simulink model "generate_joint_position_motion"  (R2021a)
settings: Solver=FixedStepDiscrete  StartTime=0.0  StopTime=inf  FixedStep=0.001  RelTol=1e-3  EnableMultiTasking=on
PreLoadFcn:
  | demos_common_configs();
libraries: franka_simulink_library x5, franka_simulink_library_misc x5
settings Model: SimulationMode=external  ExtModeTrigDuration=10000  Creator=vasi_ko  LastModifiedBy=kvasios
settings SolverCC: AlgebraicLoopSolver=TrustRegion
settings DataIOCC: LimitDataPoints=on  SaveFormat=Array  ReturnWorkspaceOutputs=off
settings OptimizationCC: DefaultParameterBehavior=Inlined  EnhancedBackFolding=on  PassReuseOutputArgsAs=Individual arguments  ZeroExternalMemoryAtStartup=off  ZeroInternalMemoryAtStartup=off  OptimizeBlockOrder=speed  DifferentSizesBufferReuse=on  OptimizationCustomize=off  EfficientTunableParamExpr=on
settings DebuggingCC: SolverPrmCheckMsg=warning  ParameterTunabilityLossMsg=error  SFUnexpectedBacktrackingDiag=warning  SFNoUnconditionalDefaultTransitionDiag=warning  SFExecutionAtInitializationDiag=none  SFMachineParentedDataDiag=warning  ArithmeticOperatorsInVariantConditions=warning
settings HardwareCC: ProdBitPerLong=64  ProdHWDeviceType=Intel->x86-64 (Linux 64)
settings ModelReferenceCC: PropagateSignalLabelsOutOfModel=off
settings SFSimCC: SimUseLocalCustomCode=off  MATLABDynamicMemAlloc=off  CustomCodeUndefinedFunction=UseInterfaceOnly  SimTargetLang=C++
settings RTWCC: SystemTargetFile=franka_emika_panda.tlc  GenCodeOnly=on  TemplateMakefile=ert_default_tmf  RTWVerbose=off  RTWUseLocalCustomCode=off  Toolchain=Franka Simulink | gmake (64-bit linux)  BuildConfiguration=Faster Runs  IncludeHyperlinkInReport=on  TargetLang=C++
settings CodeAppCC: ForceParamTrailComments=on  IgnoreCustomStorageClasses=off  OperatorAnnotations=on  SimulinkDataObjDesc=on  SFDataObjDesc=on  InsertBlockDesc=on
settings STFCustomTargetCC: TargetLangStandard=C99 (ISO)  MultiwordLength=256  GenerateSampleERTMain=on  ModelReferenceCompliant=off  CombineOutputUpdateFcns=on  ERTCustomFileBanners=on  SupportNonInlinedSFcns=off  RemoveResetFunc=on  MATLABClassNameForMDSCustomization=Simulink.SoftwareTarget.ERTCustomization  CPPClassGenCompliant=on  GRTInterface=off  SystemTargetFile=franka_emika_panda.tlc
settings ERTTargetCC: TargetLangStandard=C99 (ISO)  GenerateSampleERTMain=on  ModelReferenceCompliant=off  ParMdlRefBuildCompliant=off  CompOptLevelCompliant=off  ConcurrentExecutionCompliant=off  SupportContinuousTime=on  ModelStepFunctionPrototypeControlCompliant=off  InlinedParameterPlacement=NonHierarchical  ERTCustomFileTemplate=franka_emika_panda_file_process.tlc
settings ConfigComp: CovMetricSettings=dw  CovSaveCumulativeToWorkspaceVar=on  CovSaveSingleToWorkspaceVar=on  CovExternalEMLEnable=off  CovSFcnEnable=off

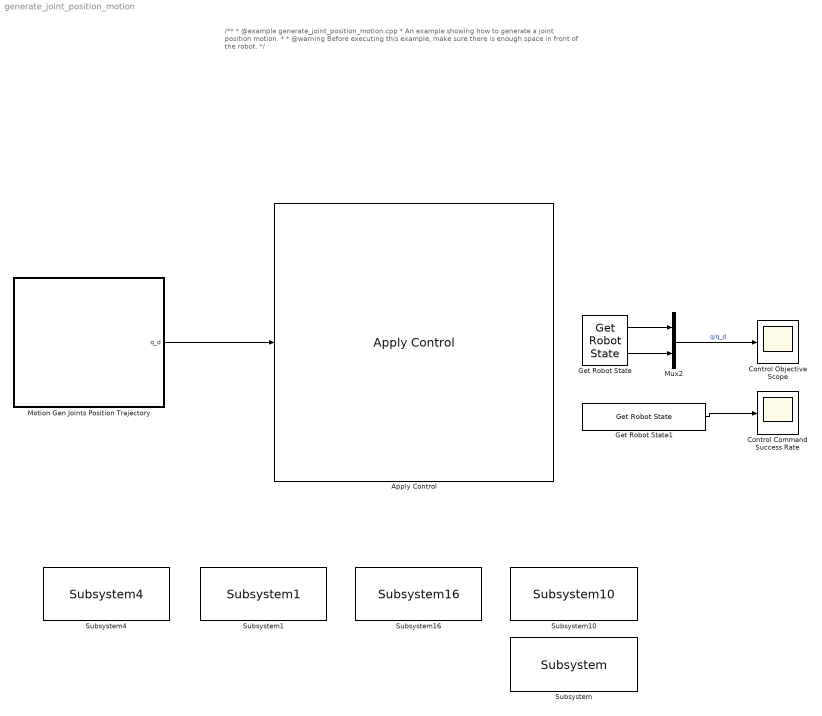
== system generate_joint_position_motion ==
  note: /**
      |  * @example generate_joint_position_motion.cpp
      |  * An example showing how to generate a joint position motion.
      |  *
      |  * @warning Before executing this example, make sure there is enough space in front of the robot.
      |  */
  Apply Control : franka_simulink_library/Apply Control  robot_ip=robot_ip  gripper_attached=off  control_mode=Joint Positions - Internal Controller Mode  controller_choice=Joint Impedance Controller  elbow_control=on  collision_thresholds=collision_behavior  joint_impedance=joint_impedance  cartesian_impedance=cartesian_impedance  load_inertia=load_inertia  EE_T_K=EE_T_K  init_joint_configuration_req=on  init_joint_configuration=q_init
      settings: SourceProductName=Franka Emika
  Control Command Success Rate : Scope
  Control Objective Scope : Scope
  Get Robot State : franka_simulink_library/Get Robot State  robot_ip=robot_ip  signals_requested='q q_d'
      settings: SourceProductName=Franka Emika
  Get Robot State1 : franka_simulink_library/Get Robot State  robot_ip=robot_ip  signals_requested='control_command_success_rate'
      settings: SourceProductName=Franka Emika
  Motion Gen Joints Position Trajectory : Subsystem
      mask Display:
      | pos = get_param(gcb, 'Position');
      | width = pos(3) - pos(1);
      | x = [0:width];
      | y = sin(x/180*pi);
      | % Parameters 'm' and 'b' must be defined in 'Parameters & Dialog' pane.
      | plot(cos(x/180*pi), sin(x/180*pi));
      | 
      | port_label('output',1,'q_d');
  Mux2 : Mux  Inputs=2
  Subsystem : franka_simulink_library_misc/Subsystem  SystemSampleTime=-1  VariantActivationTime=update diagram  Latency=0  AutoFrameSizeCalculation=off
  Subsystem1 : franka_simulink_library_misc/Subsystem1  SystemSampleTime=-1  VariantActivationTime=update diagram  Latency=0  AutoFrameSizeCalculation=off
  Subsystem10 : franka_simulink_library_misc/Subsystem10  SystemSampleTime=-1  VariantActivationTime=update diagram  Latency=0  AutoFrameSizeCalculation=off
  Subsystem16 : franka_simulink_library_misc/Subsystem16  SystemSampleTime=-1  VariantActivationTime=update diagram  Latency=0  AutoFrameSizeCalculation=off
  Subsystem4 : franka_simulink_library_misc/Subsystem4  SystemSampleTime=-1  VariantActivationTime=update diagram  Latency=0  AutoFrameSizeCalculation=off
  wires:
  Get Robot State/2 -> Mux2/2
  Mux2/1 -> Control Objective Scope/1  "q/q_d"
  Motion Gen Joints Position Trajectory/1(q_d) -> Apply Control/1
  Get Robot State/1 -> Mux2/1
  Get Robot State1/1 -> Control Command Success Rate/1

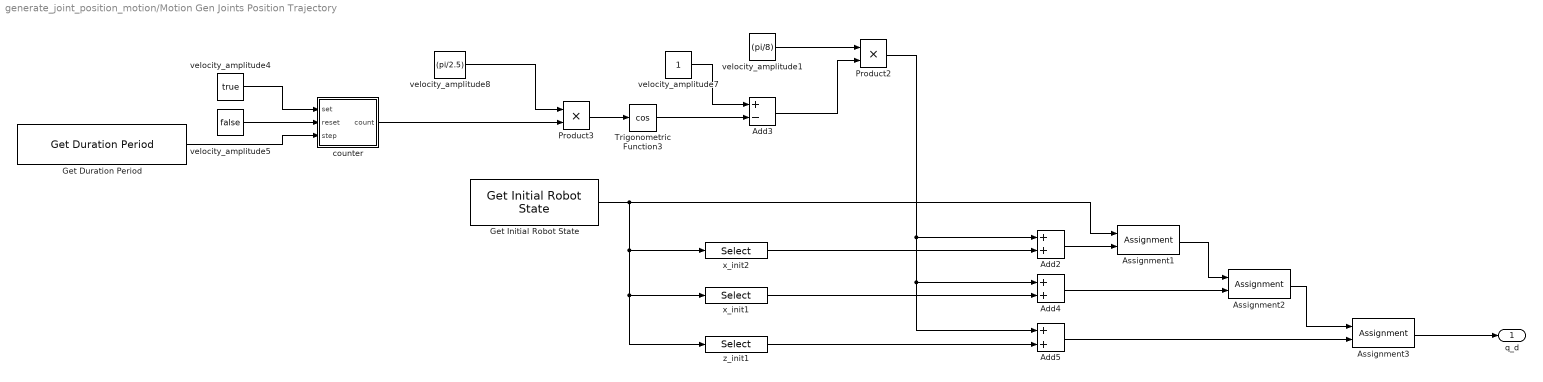
== system generate_joint_position_motion/Motion Gen Joints Position Trajectory ==
  Add2 : Sum
  Add3 : Sum  Inputs=+-
  Add4 : Sum
  Add5 : Sum
  Assignment1 : Assignment  DiagnosticForDimensions=Warning  IndexOptions=Index vector (dialog)  Indices=4  OutputSizes=1
  Assignment2 : Assignment  DiagnosticForDimensions=Warning  IndexOptions=Index vector (dialog)  Indices=5  OutputSizes=1
  Assignment3 : Assignment  DiagnosticForDimensions=Warning  IndexOptions=Index vector (dialog)  Indices=7  OutputSizes=1
  Get Duration Period : franka_simulink_library/Get Duration Period  robot_ip=robot_ip
      settings: SourceProductName=Franka Emika
  Get Initial Robot State : franka_simulink_library/Get Initial Robot State  robot_ip=robot_ip  signals_requested='q_d'
      settings: SourceProductName=Franka Emika
  Product2 : Product
  Product3 : Product
  Trigonometric Function3 : Trigonometry  Operator=cos
  counter : Subsystem
  velocity_amplitude1 : Constant  Value=(pi/8)  VectorParams1D=off
  velocity_amplitude4 : Constant  Value=true  VectorParams1D=off
  velocity_amplitude5 : Constant  Value=false  VectorParams1D=off
  velocity_amplitude7 : Constant  VectorParams1D=off
  velocity_amplitude8 : Constant  Value=(pi/2.5)  VectorParams1D=off
  x_init1 : Selector  InputPortWidth=7  IndexOptions=Index vector (dialog)  Indices=5  OutputSizes=1
  x_init2 : Selector  InputPortWidth=7  IndexOptions=Index vector (dialog)  Indices=4  OutputSizes=1
  z_init1 : Selector  InputPortWidth=7  IndexOptions=Index vector (dialog)  Indices=7  OutputSizes=1
  q_d : Outport  VectorParamsAs1DForOutWhenUnconnected=off
  wires:
  Add5/1 -> Assignment3/2
  Get Initial Robot State/1 -> z_init1/1, x_init1/1, x_init2/1, Assignment1/1
  Add4/1 -> Assignment2/2
  Assignment2/1 -> Assignment3/1
  z_init1/1 -> Add5/2
  x_init1/1 -> Add4/2
  Add2/1 -> Assignment1/2
  Assignment1/1 -> Assignment2/1
  x_init2/1 -> Add2/2
  velocity_amplitude1/1 -> Product2/1
  velocity_amplitude7/1 -> Add3/1
  Add3/1 -> Product2/2
  Product2/1 -> Add5/1, Add4/1, Add2/1
  Trigonometric Function3/1 -> Add3/2
  velocity_amplitude8/1 -> Product3/1
  Product3/1 -> Trigonometric Function3/1
  Assignment3/1 -> q_d/1
  Get Duration Period/1 -> counter/3(step)
  velocity_amplitude4/1 -> counter/1(set)
  velocity_amplitude5/1 -> counter/2(reset)
  counter/1(count) -> Product3/2

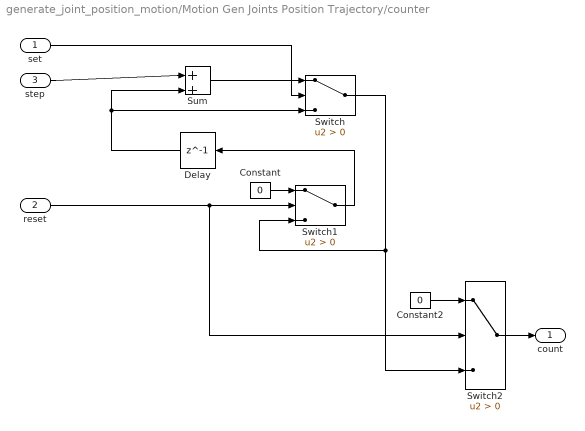
== system generate_joint_position_motion/Motion Gen Joints Position Trajectory/counter ==
  set : Inport  OutDataTypeStr=boolean
  reset : Inport  Port=2  OutDataTypeStr=boolean
  step : Inport  Port=3  OutDataTypeStr=double
  Constant : Constant  Value=0  OutDataTypeStr=double
  Constant2 : Constant  Value=0  OutDataTypeStr=double
  Delay : Delay  DelayLength=1  InitialCondition=0
  Sum : Sum  Inputs=|++
  Switch : Switch  Criteria=u2 > Threshold
  Switch1 : Switch  Criteria=u2 > Threshold  OutDataTypeStr=double
  Switch2 : Switch  Criteria=u2 > Threshold  OutDataTypeStr=double
  count : Outport  OutDataTypeStr=double  VectorParamsAs1DForOutWhenUnconnected=off
  wires:
  Switch2/1 -> count/1
  Constant2/1 -> Switch2/1
  Sum/1 -> Switch/1
  set/1 -> Switch/2
  Switch/1 -> Switch1/3, Switch2/3
  step/1 -> Sum/1
  Delay/1 -> Sum/2, Switch/3
  reset/1 -> Switch1/2, Switch2/2
  Constant/1 -> Switch1/1
  Switch1/1 -> Delay/1
